simulink model "UNCCModel"  (R2018b)
settings: Solver=ode4  StartTime=0.0  StopTime=Inf  FixedStep=0.025  RelTol=1e-3  EnableMultiTasking=on
PreLoadFcn:
  | preLoadCallback
StartFcn:
  | startCallback
StopFcn:
  | stopCallback
model workspace (MAT data in the model file):
  Ts = 0.025
undefined symbols (not defined in the file or in its folder): acA2000, Ace, Basler, Freerun_FIX_YAW, PoCL
libraries: slrtlib x3, xpcbitflowlib x3, xpcvideoutillib x2, xpcobsoletelib x1, xpcrtudplib x1
(part 1 of 3)
settings Model: xpc_rtwmakecfg_data=_jpeg__bitflow_  sg_rtwmakecfg_data=_bitflow_  SimulationMode=external  Creator=gweast  LastModifiedBy=MAE-NCSUCORE
settings DataIOCC: MaxDataPoints=40*60*60  SaveFormat=Array  SignalLoggingSaveFormat=ModelDataLogs  SignalLogging=off  DSMLogging=off  VisualizeSimOutput=off
settings OptimizationCC: BlockReduction=off  OptimizeBlockIOStorage=off  BufferReuse=off  GlobalBufferReuse=off  ExpressionFolding=off  ExpressionDepthLimit=2147483647  LocalBlockOutputs=off  LifeSpan=inf  SimCompilerOptimization=on  OptimizeDataStoreBuffers=off  BusAssignmentInplaceUpdate=off
settings DebuggingCC: UnderspecifiedInitializationDetection=Classic  MergeDetectMultiDrivingBlocksExec=none  SolverPrmCheckMsg=warning  InheritedTsInSrcMsg=none  FcnCallInpInsideContextMsg=warning  AllowSymbolicDim=off  StateNameClashWarn=warning  LibraryContextMissingDiagnostic=none  SFUnexpectedBacktrackingDiag=warning  SFNoUnconditionalDefaultTransitionDiag=warning  SFExecutionAtInitializationDiag=none
settings HardwareCC: ProdBitPerPointer=32  ProdBitPerSizeT=32  ProdBitPerPtrDiffT=32  ProdLargestAtomicFloat=None  ProdWordSize=32  ProdLongLongMode=on  ProdHWDeviceType=Generic->32-bit x86 compatible  TargetBitPerLong=64  TargetBitPerPointer=64  TargetIntDivRoundTo=Zero  TargetEndianess=LittleEndian  TargetWordSize=64  TargetHWDeviceType=Intel->x86-64
settings ModelReferenceCC: UpdateModelReferenceTargets=Force  PropagateSignalLabelsOutOfModel=off
settings SFSimCC: SimUseLocalCustomCode=off
settings RTWCC: SystemTargetFile=slrt.tlc  TLCOptions=-axPCModelStackSizeKB=512  TemplateMakefile=slrt_default_tmf  Description=Simulink Real-Time  GenerateReport=on  RTWUseLocalCustomCode=off  CodeExecutionProfiling=on  RTWCompilerOptimization=on
settings CodeAppCC: StateflowObjectComments=on
settings SimulinkRealTimeCC: PreserveStateflowLocalDataDimensions=off  RL32LogBufSizeModifier=32400000  xPCRL32EventNumber=50000  xPCisModelTimeout=off  xPCModelTimeoutSecs=30
settings ConfigComp: CovMetricSettings=dw  CovHtmlReporting=on  CovSaveCumulativeToWorkspaceVar=on  CovSaveSingleToWorkspaceVar=on  CovExternalEMLEnable=off

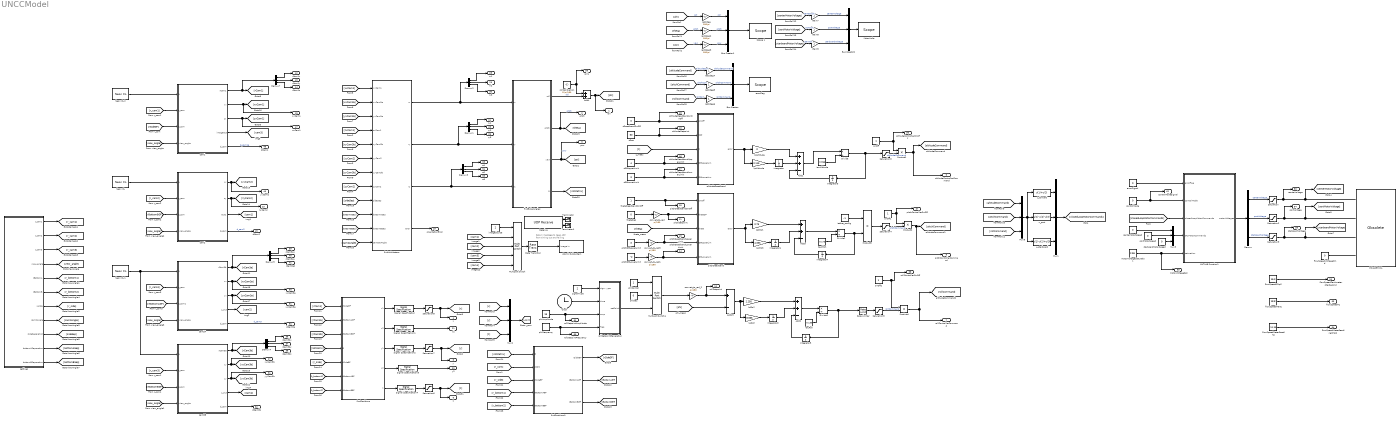
== system UNCCModel ==
  note: Return message to keep ARP
      | from timing out and failing
  Add1 : Sum  Inputs=++-
  Add19 : Sum  Inputs=+-
  Add2 : Sum  Inputs=++-
  Add3 : Sum  Inputs=++-
  Add4 : Sum
  Atomic Subsystem : Subsystem  TreatAsAtomicUnit=on  SystemSampleTime=Ts*3
  Bus Creator : BusCreator  Inputs=3
  Bus Creator1 : BusCreator  Inputs=3
  Bus Creator2 : BusCreator  Inputs=3
  Clock : Clock
  Demux{,1..5,7} (7 alike) : Demux  Outputs=3
  Divide : Product  Inputs=*/
  Divide1 : Product  Inputs=*/
  Divide2 : Product  Inputs=*/
  Gain7 : Gain
  Gain8 : Gain
  Gain9 : Gain
  Integrator{,1..5} (6 alike) : Integrator  InitialCondition=0.001
  MATLAB Function1 : MATLAB Function  TreatAsAtomicUnit=on
  "MotorVolts " : slrtlib/Displays and Logging/Scope   Tag=Motor Volts  Priority=2  scopeno=2  scopetype=Target  autostart=on  viewmode=Graphical rolling  formatstr='%15.6f'  grid=on  ylimits=[0,4]  nosamples=400  noprepostsamples=0  interleave=1  triggermode=FreeRun  triggersignal=1  trigsignalfromport=off  triggerlevel=0.0  triggerslope=Either  triggerscope=1  triggersample=0  filename=data.dat  mode=Lazy  writesize=512  autorestart=off  dynamicfilemode=off  maxwritefilesize=512*1024^2
  Multiport Switch : MultiPortSwitch  DataPortOrder=Zero-based contiguous  Inputs=4  zeroidx=on
  Multiport Switch4 : MultiPortSwitch  Inputs=2
  Mux{1..3,8} (4 alike) : Mux  Inputs=3
  "Neon CL " : xpcbitflowlib/Neon CL   camerapath=Basler-Ace-acA2000-340km-PoCL-3Tap-Freerun_FIX - ROLL.r64  r64=CAMERA  sampletime=-1  slot=[7,12]  make=Basler  model=acA2000-340km  mode=3 tap, 8-bits, 2040x1088 PoCL Free running  owner=BitFlow  revision=1  modelcomp=0  revcomp=0  aqtimeout=61440  format=1  flashmux=Mux_2TOEP  flashdcc=DCC  pixbitdepth=8  xsize=2040  ysize=1088  xstart=0  ystart=0  dx=2040  dy=1088  expmod="[0  0]"  config="[4294967295         128;4294967295           0;4294967295         512;4294967295           0;4294967295           0;4294967295           0;4294967295      262144;4294967295           0;4294967295           0;4294967295           0;4294967295     4195324;4294967295           0;4294967295           0;4294967295  4294967295;4294967295           0;4294967295           0;4294967295           0;4294967295    16777215;4294967295        1088;4294967295           0;4294967295           0;4294967295    16777215;4294967295           0;4294967295           0;4294967295           0;4294967295           0;4294967295           0;4294967295           0]"  ctab="[6      0     16      1  36880      2     16     96     18     97     16  32768      0]"  qtabmodel="[1   2040  65536]"  trigmode=0  baud=1  bytewidth=4  parity=1  stopbits=1  command="\"\""  response=0  comments=|
      | Three tap camera, 
      | Acquistion acquires 24 bits per clock, 
      | DMA works as 8-bit data
      | Set XSIZE = 3 * ACPL
      settings: SourceProductName=Simulink Real-Time: Speedgoat I/O Driver Library
  Neon CL 1 : xpcbitflowlib/Neon CL   camerapath=Basler-Ace-acA2000-340km-PoCL-3Tap-Freerun_FIX_YAW.r64  r64=CAMERA  sampletime=-1  slot=[4,12]  make=Basler  model=acA2000-340km  mode=3 tap, 8-bits, 2040x1088 PoCL Free running  owner=BitFlow  revision=1  modelcomp=0  revcomp=0  aqtimeout=61440  format=1  flashmux=Mux_2TOEP  flashdcc=DCC  pixbitdepth=8  xsize=2040  ysize=1088  xstart=0  ystart=0  dx=2040  dy=1088  expmod="[0  0]"  config="[4294967295         128;4294967295           0;4294967295         512;4294967295           0;4294967295           0;4294967295           0;4294967295      262144;4294967295           0;4294967295           0;4294967295           0;4294967295     4195324;4294967295           0;4294967295           0;4294967295  4294967295;4294967295           0;4294967295           0;4294967295           0;4294967295     4958209;4294967295        1088;4294967295           0;4294967295           0;4294967295  2164260863;4294967295           0;4294967295           0;4294967295           0;4294967295           0;4294967295     4958208;4294967295           0]"  ctab="[6      0     16      1  36880      2     16     96     18     97     16  32768      0]"  qtabmodel="[1   2040  65536]"  trigmode=0  baud=1  bytewidth=4  parity=1  stopbits=1  command="\"\""  response=0  comments=|
      | Three tap camera, 
      | Acquistion acquires 24 bits per clock, 
      | DMA works as 8-bit data
      | Set XSIZE = 3 * ACPL
      settings: SourceProductName=Simulink Real-Time: Speedgoat I/O Driver Library
  Neon CL 2 : xpcbitflowlib/Neon CL   camerapath=Basler-Ace-acA2000-340km-PoCL-3Tap-Freerun_FIX - PITCH.r64  r64=CAMERA  sampletime=-1  slot=[13,12]  make=Basler  model=acA2000-340km  mode=3 tap, 8-bits, 2040x1088 PoCL Free running  owner=BitFlow  revision=1  modelcomp=0  revcomp=0  aqtimeout=61440  format=1  flashmux=Mux_2TOEP  flashdcc=DCC  pixbitdepth=8  xsize=2040  ysize=1088  xstart=0  ystart=0  dx=2040  dy=1088  expmod="[0  0]"  config="[4294967295         128;4294967295           0;4294967295         512;4294967295           0;4294967295           0;4294967295           0;4294967295      262144;4294967295           0;4294967295           0;4294967295           0;4294967295     4195324;4294967295           0;4294967295           0;4294967295  4294967295;4294967295           0;4294967295           0;4294967295           0;4294967295     7528449;4294967295        1088;4294967295           0;4294967295           0;4294967295           0;4294967295           0;4294967295           0;4294967295           0;4294967295           0;4294967295     7528448;4294967295           0]"  ctab="[6      0     16      1  36880      2     16     96     18     97     16  32768      0]"  qtabmodel="[1   2040  65536]"  trigmode=0  baud=1  bytewidth=4  parity=1  stopbits=1  command="\"\""  response=0  comments=|
      | Three tap camera, 
      | Acquistion acquires 24 bits per clock, 
      | DMA works as 8-bit data
      | Set XSIZE = 3 * ACPL
      settings: SourceProductName=Simulink Real-Time: Speedgoat I/O Driver Library
  PCI-6259 DA : xpcobsoletelib/Obsolete
      settings: SourceProductName=Simulink Real-Time  SourceProductBaseCode=XP
  Product{1..4} (4 alike) : Product
  Rate Limiter : RateLimiter  RisingSlewLimit=20  FallingSlewLimit=-20  SampleTimeMode=inherited
  Rate Transition : RateTransition
  Receive : xpcrtudplib/UDP Receive  ipAddressVal=Use host-target connection  localPort=25005  rcvWidth=1  rcvFmAny=off  fmAddress=10.10.10.10  rcvMulticast=off  multicastAddress=[]  maxUDPQueue=8  sampleTime=-1
      settings: SourceProductName=Simulink Real-Time
  Saturation : Saturate  UpperLimit=3.3  LowerLimit=0
  Saturation2 : Saturate  UpperLimit=3.3  LowerLimit=0
  Saturation3 : Saturate  UpperLimit=1.65  LowerLimit=-1.65
  Saturation4 : Saturate  UpperLimit=1.65  LowerLimit=-1.65
  Saturation5 : Saturate  UpperLimit=1.65  LowerLimit=-1.65
  Saturation6 : Saturate  UpperLimit=90  LowerLimit=10
  Saturation7 : Saturate  UpperLimit=50  LowerLimit=-50
  Saturation8 : Saturate  UpperLimit=100  LowerLimit=-10
  Saturation9 : Saturate  UpperLimit=3.3  LowerLimit=0
  Scope 1 : slrtlib/Displays and Logging/Scope   scopeno=1  scopetype=Target  autostart=on  viewmode=Graphical rolling  formatstr='%15.6f'  grid=on  ylimits=[-45,45]  nosamples=400  noprepostsamples=0  interleave=1  triggermode=FreeRun  triggersignal=1  trigsignalfromport=off  triggerlevel=0.0  triggerslope=Either  triggerscope=1  triggersample=0  filename=data.dat  mode=Lazy  writesize=512  autorestart=off  dynamicfilemode=off  maxwritefilesize=512*1024^2
  Signal Specification{,1..4} (5 alike) : SignalSpecification  Dimensions=1
  Terminator : Terminator
  Terminator1 : Terminator
  altitudeDeadband : MATLAB Function  TreatAsAtomicUnit=on
  cam1 : Subsystem
  cam2 : Subsystem
  cam3A : Subsystem
  cam3B : Subsystem
  centerMotorSpeed : Constant  Value=0
  controlMode : Constant  Value=0
  convert_to_rad : Gain  Gain=pi/180
  convert_to_rad1 : Gain  Gain=pi/180
  convert_to_rad3 : Gain  Gain=pi/180
  convert_to_rad_2 : Gain  Gain=pi/180
  errorFlag : slrtlib/Displays and Logging/Scope   Tag=Motor Volts  Priority=2  scopeno=4  scopetype=Target  autostart=on  viewmode=Graphical rolling  formatstr='%15.6f'  grid=on  ylimits=[-2,2]  nosamples=400  noprepostsamples=0  interleave=1  triggermode=FreeRun  triggersignal=1  trigsignalfromport=off  triggerlevel=0.0  triggerslope=Either  triggerscope=1  triggersample=0  filename=data.dat  mode=Lazy  writesize=512  autorestart=off  dynamicfilemode=off  maxwritefilesize=512*1024^2
  errorSignal : Constant  Value=0
  findEulerAngles : MATLAB Function  TreatAsAtomicUnit=on
  findPositions : MATLAB Function  TreatAsAtomicUnit=on
  findPositions1 : MATLAB Function  TreatAsAtomicUnit=on
  findUnitVectors : MATLAB Function  TreatAsAtomicUnit=on
  flowSpeedCMpS : Constant  Value=16.3
  flowSpeedHertz : Constant  Value=18.8
  flowSpeedMeterReading : Constant  Value=20.39
  flowSpeedVoltageCmd : Constant  Value=0
  imageSource : Constant  Value=2
  kdAltitude : Gain  Gain=0
  kdPitch : Gain  Gain=0.75
  kdRoll : Gain  Gain=2.250
  kpAltitude : Gain  Gain=0.115
  kpPitch : Gain  Gain=4.333
  kpRoll : Gain  Gain=8.666
  motorVoltageSaturation : Constant  Value=2.56
  onOff : Constant
  onOff1 : Constant
  onOff2 : Constant
  phiAmplitude : Constant  Value=15
  phiControl : Constant
  phiDes : Constant  Value=0
  phiFrequency : Constant  Value=1/6.875
  pitchDBLowerLimit : Constant  Value=-2
  pitchDBUpperLimit : Constant  Value=3
  pitchDeadband : MATLAB Function  TreatAsAtomicUnit=on
  portMotorSpeed : Constant  Value=0
  rad2deg : Gain  Gain=180/pi
  rad2deg2 : Gain  Gain=180/pi
  rad2deg3 : Gain  Gain=180/pi
  rad2deg4 : Gain
  "rad2deg5 " : Gain
  rad2deg6 : Gain
  rollCalibration : Constant  Value=5*pi/180
  rollSetpointGeneration : MATLAB Function  TreatAsAtomicUnit=on
  settings : Subsystem
  signalType : Constant  Value=2
  starboardMotorSpeed : Constant  Value=0
  tauAltitude : Constant  Value=0.866
  tauPitch : Constant  Value=0.173
  tauRoll : Constant  Value=0.130
  tether_config : Constant  Value=-1
  thetaDeadbandOnOff : Constant
  thetaDes : Constant  Value=0
  u_forward : Fcn  Expr=u(1)+u(2)
  u_port : Fcn  Expr=u(1)-u(2)-u(3)
  u_starboard : Fcn  Expr=u(1)-u(2)+u(3)
  zDBLowerLimit : Constant  Value=3
  zDBUpperLimit : Constant  Value=4
  zDeadbandOnOff : Constant  Value=0
  zDes : Constant  Value=50
  roll : Outport
  pitch : Outport  Port=2
  yaw : Outport  Port=3
  x : Outport  Port=4
  y : Outport  Port=5
  z : Outport  Port=6
  rollControllerCommand : Outport  Port=7
  pitchControllerCommand : Outport  Port=8
  altitudeControllerCommand : Outport  Port=9
  altitudeSetpoint : Outport  Port=10
  pitchSetpoint : Outport  Port=11
  rollSetpoint : Outport  Port=12
  pitchDeadbandUpperLimit : Outport  Port=13
  pitchDeadbandLowerLimit : Outport  Port=14
  pitchDeadbandOnOff : Outport  Port=15
  altitudeDeadbandUpperLimit : Outport  Port=16
  altitudeDeadbandLowerLimit : Outport  Port=17
  altitudeDeadbandonOnOff : Outport  Port=18
  orientationError : Outport  Port=19
  flowSpeedCentimetersPerSecond : Outport  Port=20
  x2 : Outport  Port=21
  y2 : Outport  Port=22
  zyCam2 : Outport  Port=23
  ry1 : Outport  Port=24
  ry2 : Outport  Port=25
  ry3 : Outport  Port=26
  xyCam3b : Outport  Port=27
  rx1 : Outport  Port=28
  rx2 : Outport  Port=29
  rx3 : Outport  Port=30
  yyCam3b : Outport  Port=31
  dCam3b : Outport  Port=32
  rz1 : Outport  Port=33
  rz2 : Outport  Port=34
  rz3 : Outport  Port=35
  rCam3bx : Outport  Port=36
  rCam3by : Outport  Port=37
  rCam3bz : Outport  Port=38
  rCam3ax : Outport  Port=39
  rCam3ay : Outport  Port=40
  rCam3az : Outport  Port=41
  rCam1x : Outport  Port=42
  rCam1y : Outport  Port=43
  rCam1z : Outport  Port=44
  yyCam2 : Outport  Port=45
  xxCam1 : Outport  Port=46
  zxCam1 : Outport  Port=47
  dCam1 : Outport  Port=48
  dCam2 : Outport  Port=49
  xxCam3a : Outport  Port=50
  yxCam3a : Outport  Port=51
  dCam3a : Outport  Port=52
  centerVoltage : Outport  Port=53
  portVoltage : Outport  Port=54
  starboardVoltage : Outport  Port=55
  altitudeControllerOnOff : Outport  Port=56
  pitchControllerOnOff : Outport  Port=57
  rollControllerOnOff : Outport  Port=58
  roll1 : Outport  Port=59
  rollSetpointFrequency : Outport  Port=60
  rollSetpointAmplitude : Outport  Port=61
  controlModeSignal : Outport  Port=62
  flowSpeedHz : Outport  Port=63
  flowSpeedMeterReadingCMpS : Outport  Port=64
  motorVoltageSat : Outport  Port=65
  wires:
  controlMode/1 -> controlModeSignal/1, MATLAB Function1/2(controlMode)
  [phi] -> Add19/2
  [theta] -> pitchDeadband/3(theta)
  cam1/1(rCam1) -> [rCam1], Demux7/1
  cam3A/1(rCam3b) -> Demux5/1, [rCam3a]
  Demux/3 -> Saturation9/1  "starboardVoltage"
  Neon CL 1/1 -> cam3B/1("u "), cam3A/1(u)
  cam1/2(xx) -> xxCam1/1, [xxCam1]
  cam1/3(zx) -> zxCam1/1, [zxCam1]
  cam3A/3(yx) -> yxCam3a/1, [yxCam3a]
  findEulerAngles/2(pitch) -> [theta], pitch/1  "pitch"
  findEulerAngles/3(yaw) -> [psi], yaw/1  "yaw"
  convert_to_rad_2/1 -> Add19/1, rollSetpoint/1
  tether_config/1 -> Product3/1
  Product3/1 -> Saturation4/1
  cam3B/2(xy) -> xyCam3b/1, [xyCam3b]
  cam3B/3(yy) -> yyCam3b/1, [yyCam3b]
  cam2/1(yy) -> yyCam2/1, [yyCam2]
  cam2/2(zy) -> zyCam2/1, [zyCam2]
  Neon CL 2/1 -> cam1/1("u ")
  cam3B/4(u_out) -> [cam4]
  cam2/3(Out1) -> [cam1]
  "Neon CL "/1 -> cam2/1("u ")
  cam3A/4("u_out ") -> [cam2]
  settings/1(r_cam1) -> [r_cam1]
  settings/2("r_cam2 ") -> [r_cam2]
  settings/3(r_cam3) -> [r_cam3]
  [r_cam1] -> cam1/2(r_cam)
  [r_cam3] -> cam3B/2(r_cam)
  [r_cam2] -> cam2/2(r_cam)
  [r_cam3] -> cam3A/2(r_cam)
  [rBottomBGF] -> cam3B/3("r_com ")
  [rBottomBGF] -> cam2/3("r_com ")
  [rBottomAGF] -> cam3A/3(r_com1)
  [rSideGF] -> cam1/3("r_com ")
  cam3B/5(d_cam) -> dCam3b/1
  settings/4(view_angle) -> [view_angle]
  [view_angle] -> cam1/4(view_angle)
  [view_angle] -> cam3B/4(view_angle)
  [view_angle] -> cam2/4(view_angle)
  [view_angle] -> cam3A/4(view_angle)
  cam1/4(imageOut) -> [cam3]
  phiAmplitude/1 -> rollSetpointAmplitude/1, rollSetpointGeneration/3(amp)
  phiFrequency/1 -> rollSetpointFrequency/1, rollSetpointGeneration/4(freq)
  Multiport Switch4/1 -> convert_to_rad_2/1
  rollSetpointGeneration/1(setPoint) -> Multiport Switch4/3
  phiDes/1 -> Multiport Switch4/2
  phiControl/1 -> Multiport Switch4/1
  thetaDes/1 -> convert_to_rad/1
  Clock/1 -> rollSetpointGeneration/2(time)
  portMotorSpeed/1 -> Mux3/2
  Mux3/1 -> MATLAB Function1/4(GUIMotorCommands)
  signalType/1 -> rollSetpointGeneration/1(signalType)
  Rate Limiter/1 -> Saturation5/1
  zDes/1 -> altitudeDeadband/2(zSP), altitudeSetpoint/1
  u_forward/1 -> Mux1/1
  u_port/1 -> Mux1/2
  u_starboard/1 -> Mux1/3
  [closedLoopMotorCommands] -> MATLAB Function1/3(closedLoopMotorCommands)
  centerMotorSpeed/1 -> Mux3/1
  starboardMotorSpeed/1 -> Mux3/3
  [psi] -> rad2deg3/1  "yaw"
  [theta] -> rad2deg2/1  "pitch"
  [phi] -> rad2deg/1  "roll"
  [z] -> Mux2/3
  [y] -> Mux2/2
  [x] -> Mux2/1
  Saturation6/1 -> z/1, [z]
  Saturation7/1 -> [y], y/1
  Saturation8/1 -> x/1, [x]
  [rollCommand] -> Mux8/3
  [pitchCommand] -> Mux8/2
  [altitudeCommand] -> Mux8/1
  Divide/1 -> Integrator3/1, Saturation3/1
  Divide1/1 -> Integrator4/1, Product3/2
  MATLAB Function1/1(motorVoltages) -> Demux/1
  Demux/2 -> Saturation2/1  "portVoltage"
  Demux/1 -> Saturation/1  "centerVoltage"
  Bus Creator2/1 -> "MotorVolts "/1
  settings/5(rBottomA) -> [r_bottom1]
  settings/7(r_side) -> [r_side]
  convert_to_rad/1 -> pitchSetpoint/1, pitchDeadband/2(thetaSP)
  pitchDBUpperLimit/1 -> convert_to_rad3/1
  convert_to_rad3/1 -> pitchDeadband/4(DBUpperLim), pitchDeadbandUpperLimit/1
  errorSignal/1 -> MATLAB Function1/1(errorFlag)
  pitchDBLowerLimit/1 -> convert_to_rad1/1
  convert_to_rad1/1 -> pitchDeadband/5(DBLowerLim), pitchDeadbandLowerLimit/1
  thetaDeadbandOnOff/1 -> pitchDeadbandOnOff/1, pitchDeadband/1(onOff)
  [z] -> altitudeDeadband/3(z)
  zDeadbandOnOff/1 -> altitudeDeadbandonOnOff/1, altitudeDeadband/1(onOff)
  zDBUpperLimit/1 -> altitudeDeadbandUpperLimit/1, altitudeDeadband/4(DBUpperLim)
  zDBLowerLimit/1 -> altitudeDeadbandLowerLimit/1, altitudeDeadband/5(DBLowerLim)
  [zyCam2] -> findUnitVectors/8(zyCam2)
  [xxCam1] -> findUnitVectors/1(xxCam1)
  [zxCam1] -> findUnitVectors/4(zxCam1)
  [xxCam3a] -> findUnitVectors/2(xxCam3a)
  [xyCam3b] -> findUnitVectors/5(xyCam3b)
  [yxCam3a] -> findUnitVectors/3(yxCam3a)
  [yyCam3b] -> findUnitVectors/7(yyCam3b)
  [yyCam2] -> findUnitVectors/6(yyCam2)
  [cam2Angle] -> findUnitVectors/12(cameraAngle)
  settings/8(cam2Angle) -> [cam2Angle]
  findUnitVectors/4(error) -> orientationError/1
  settings/6(rBottomB) -> [r_bottom2]
  cam3B/1(rCam3a) -> Demux4/1, [rCam3b]
  [rCam1] -> findPositions/1(rSideGF)
  [rCam3a] -> findPositions/2(rBottomAGF)
  [rCam3b] -> findPositions/3(rBottomBGF)
  [r_side] -> findPositions/5(rSideBF)
  [r_bottom1] -> findPositions/6(rBottomABF)
  [r_bottom2] -> findPositions/7(rBottomBBF)
  [bottomBSep] -> findUnitVectors/11(bottomBSep)
  [bottomASep] -> findUnitVectors/10(bottomASep)
  [sideSep] -> findUnitVectors/9(sideSep)
  settings/9(sideSeparation) -> [sideSep]
  settings/10(bottomASeparation) -> [bottomASep]
  settings/11(bottomBSeparation) -> [bottomBSep]
  [rotMatrix] -> findPositions/4(R)
  Rate Transition/1 -> Atomic Subsystem/1(Image In)
  Receive/1 -> Terminator/1
  Receive/2 -> Terminator1/1
  imageSource/1 -> Multiport Switch/1
  [cam1] -> Multiport Switch/2
  [cam3] -> Multiport Switch/4
  [cam2] -> Multiport Switch/3
  Multiport Switch/1 -> Rate Transition/1
  [cam4] -> Multiport Switch/5
  findEulerAngles/4(R) -> [rotMatrix]
  flowSpeedCMpS/1 -> flowSpeedCentimetersPerSecond/1
  kpAltitude/1 -> Integrator/1
  altitudeDeadband/1(error) -> kpAltitude/1, kdAltitude/1
  kdAltitude/1 -> Add1/1
  Integrator/1 -> Add1/2
  Add1/1 -> Divide/1
  tauAltitude/1 -> Divide/2
  Integrator3/1 -> Add1/3
  cam1/5(d_cam) -> dCam1/1  "d_cam1a"
  cam2/4(d_cam) -> dCam2/1  "d_cam2"
  cam3A/5(d_cam) -> dCam3a/1  "d_cam3"
  Bus Creator1/1 -> Scope 1/1
  Mux1/1 -> [closedLoopMotorCommands]
  pitchDeadband/1(error) -> kdPitch/1, kpPitch/1
  kpPitch/1 -> Integrator1/1
  Integrator1/1 -> Add3/2
  kdPitch/1 -> Add3/1
  Add3/1 -> Divide1/1
  tauPitch/1 -> Divide1/2
  Integrator4/1 -> Add3/3
  Add19/1 -> kpRoll/1, kdRoll/1
  kpRoll/1 -> Integrator2/1
  Integrator2/1 -> Add2/2
  kdRoll/1 -> Add2/1
  Add2/1 -> Divide2/1
  tauRoll/1 -> Divide2/2
  Integrator5/1 -> Add2/3
  Divide2/1 -> Integrator5/1, Rate Limiter/1
  Mux8/1 -> u_starboard/1, u_forward/1, u_port/1
  Bus Creator/1 -> errorFlag/1
  findPositions/1(x1) -> Signal Specification/1
  findPositions/5(z) -> Signal Specification4/1
  findPositions/3(y1) -> Signal Specification2/1
  findPositions/2(x2) -> Signal Specification1/1
  findPositions/4(y2) -> Signal Specification3/1
  rad2deg/1 -> Bus Creator1/1  "roll"
  rad2deg2/1 -> Bus Creator1/2  "pitch"
  rad2deg3/1 -> Bus Creator1/3  "yaw"
  [altitudeCommand] -> rad2deg4/1  "altitudeCom"
  [pitchCommand] -> "rad2deg5 "/1  "pitchCom"
  [rollCommand] -> rad2deg6/1  "rollCom"
  rad2deg4/1 -> Bus Creator/1  "altitudeCommand"
  "rad2deg5 "/1 -> Bus Creator/2  "pitchCommand"
  rad2deg6/1 -> Bus Creator/3  "rollCommand"
  [centerMotorVoltage] -> Gain7/1  "centerVolt"
  [portMotorVoltage] -> Gain8/1  "portVolt"
  [starboardMotorVoltage] -> Gain9/1  "starVolt"
  Gain7/1 -> Bus Creator2/1  "centerVoltage"
  Gain8/1 -> Bus Creator2/2  "portVoltage"
  Gain9/1 -> Bus Creator2/3  "starboardVoltage"
  Demux1/1 -> ry1/1
  Demux1/2 -> ry2/1
  Demux1/3 -> ry3/1
  Demux2/1 -> rx1/1
  Demux2/2 -> rx2/1
  Demux2/3 -> rx3/1
  Demux3/1 -> rz1/1
  Demux3/2 -> rz2/1
  Demux3/3 -> rz3/1
  Demux4/1 -> rCam3bx/1
  Demux4/2 -> rCam3by/1
  Demux4/3 -> rCam3bz/1
  Demux5/1 -> rCam3ax/1
  Demux5/2 -> rCam3ay/1
  Demux5/3 -> rCam3az/1
  Demux7/1 -> rCam1x/1
  Demux7/2 -> rCam1y/1
  Demux7/3 -> rCam1z/1
  cam3A/2(xx) -> xxCam3a/1, [xxCam3a]
  Saturation/1 -> centerVoltage/1, [centerMotorVoltage]
  Saturation2/1 -> portVoltage/1, [portMotorVoltage]
  Saturation9/1 -> starboardVoltage/1, [starboardMotorVoltage]
  Saturation3/1 -> Product1/2  "altitudeCommand"
  Product1/1 -> altitudeControllerCommand/1, [altitudeCommand]
  onOff/1 -> altitudeControllerOnOff/1, Product1/1
  Saturation4/1 -> Product2/2  "pitchCommand"
  Product2/1 -> pitchControllerCommand/1, [pitchCommand]
  onOff1/1 -> pitchControllerOnOff/1, Product2/1
  Saturation5/1 -> Product4/2  "rollCommand"
  Product4/1 -> rollControllerCommand/1, [rollCommand]
  onOff2/1 -> rollControllerOnOff/1, Product4/1
  [r_com] -> findPositions1/2(rCOM)
  [r_side] -> findPositions1/3(rSideBF)
  [r_bottom1] -> findPositions1/4(rBottomABF)
  [r_bottom2] -> findPositions1/5(rBottomBBF)
  findPositions1/1(rSideGF) -> [rSideGF]
  findPositions1/2(rBottomAGF) -> [rBottomAGF]
  findPositions1/3(rBottomBGF) -> [rBottomBGF]
  [rotMatrix] -> findPositions1/1(R)
  Add4/1 -> roll/1, [phi]
  findEulerAngles/1(roll) -> Add4/2  "roll"
  rollCalibration/1 -> roll1/1, Add4/1
  Signal Specification/1 -> Saturation8/1
  Signal Specification1/1 -> x2/1
  Signal Specification2/1 -> Saturation7/1
  Signal Specification3/1 -> y2/1
  Signal Specification4/1 -> Saturation6/1
  Mux2/1 -> [r_com]
  findUnitVectors/1(rx) -> Demux2/1, findEulerAngles/1(rx)
  findUnitVectors/2(ry) -> Demux1/1, findEulerAngles/2(ry)
  findUnitVectors/3(rz) -> Demux3/1, findEulerAngles/3(rz)
  motorVoltageSaturation/1 -> motorVoltageSat/1, MATLAB Function1/5(saturation)
  flowSpeedHertz/1 -> flowSpeedHz/1
  flowSpeedMeterReading/1 -> flowSpeedMeterReadingCMpS/1
  flowSpeedVoltageCmd/1 -> ?

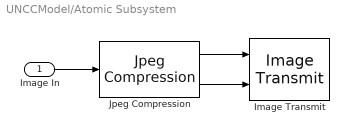
== system UNCCModel/Atomic Subsystem ==
  Image In : Inport
  Image Transmit : xpcvideoutillib/Image Transmit  ipAddress=255.255.255.255  ipPort=25000  localPort=-1  vblLen=on  maxpacket=40*1024  sampletime=-1
      settings: SourceProductName=Simulink Real-Time  SourceProductBaseCode=XP
  Jpeg Compression : xpcvideoutillib/Jpeg Compression  quality=35  cspace=Grayscale  isig=One multidimensional signal  maxsize=2040*1088  length=on
      settings: SourceProductName=Simulink Real-Time  SourceProductBaseCode=XP
  wires:
  Jpeg Compression/1 -> Image Transmit/1
  Jpeg Compression/2 -> Image Transmit/2
  Image In/1 -> Jpeg Compression/1

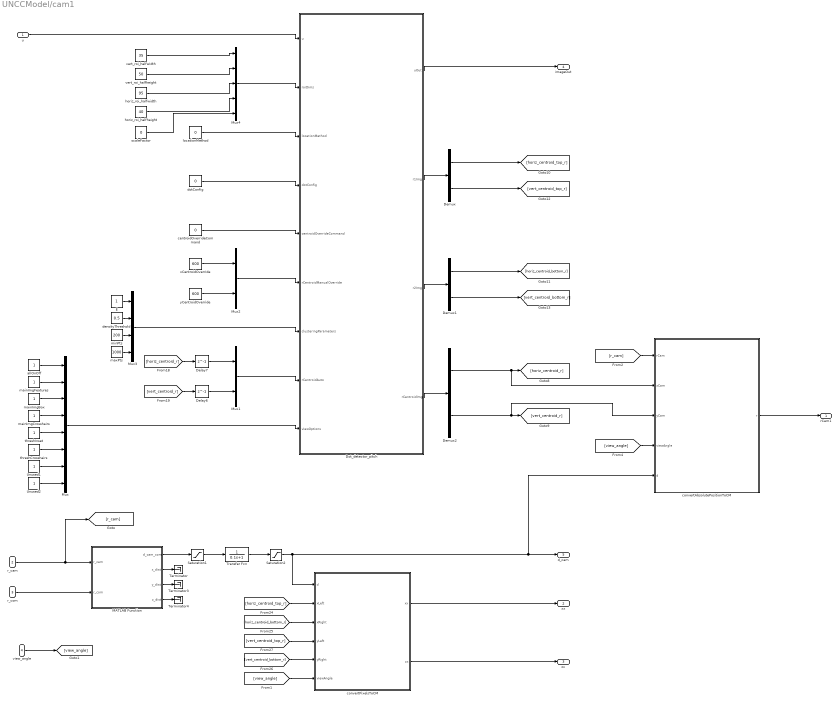
== system UNCCModel/cam1 ==
  "u " : Inport
  r_cam : Inport  Port=2
  "r_com " : Inport  Port=3
  view_angle : Inport  Port=4
  Delay6 : Delay  DelayLength=1  InitialCondition=800
  Delay7 : Delay  DelayLength=1  InitialCondition=1460
  Demux : Demux  Outputs=2
  Demux1 : Demux  Outputs=2
  Demux2 : Demux  Outputs=2
  Dot_detector_pitch : MATLAB Function  TreatAsAtomicUnit=on
  E : Constant
  MATLAB Function : MATLAB Function  TreatAsAtomicUnit=on
  Mux : Mux  Inputs=8
  Mux1 : Mux  Inputs=2
  Mux2 : Mux  Inputs=2
  Mux3 : Mux
  Mux4 : Mux  Inputs=5
  Saturation1 : Saturate  UpperLimit=200  LowerLimit=1
  Saturation2 : Saturate  UpperLimit=200  LowerLimit=1
  Terminator : Terminator
  Terminator3 : Terminator
  Terminator4 : Terminator
  Transfer Fcn : TransferFcn  Denominator=[0.1 1]
  Unused1 : Constant
  Unused2 : Constant
  allOnOff : Constant
  centroidOverrideCommand : Constant  Value=0
  convertAbsolutePositionToCM : MATLAB Function  TreatAsAtomicUnit=on
  convertPixelsToCM : MATLAB Function  TreatAsAtomicUnit=on
  densityThreshold : Constant  Value=0.5
  dotConfig : Constant  Value=0
  horiz_roi_halfheight : Constant  Value=40
  horiz_roi_halfwidth : Constant  Value=95
  locationMethod : Constant  Value=0
  mainImgBox : Constant
  mainImgCrosshairs : Constant
  mainImgFeatures : Constant
  maxPts : Constant  Value=1000
  minPts : Constant  Value=200
  scaleFactor : Constant  Value=0
  threshCrosshairs : Constant
  threshInset : Constant
  vert_roi_halfheight : Constant  Value=50
  vert_roi_halfwidth : Constant  Value=35
  xCentroidOverride : Constant  Value=600
  yCentroidOverride : Constant  Value=600
  rCam1 : Outport
  xx : Outport  Port=2
  zx : Outport  Port=3
  imageOut : Outport  Port=4
  d_cam : Outport  Port=5
  wires:
  Demux/1 -> [horiz_centroid_top_r]
  Demux1/1 -> [horiz_centroid_bottom_r]
  Demux2/2 -> convertAbsolutePositionToCM/3(yCam), [vert_centroid_r]
  Demux1/2 -> [vert_centroid_bottom_r]
  Demux/2 -> [vert_centroid_top_r]
  [horiz_centroid_r] -> Delay7/1
  [vert_centroid_r] -> Delay6/1
  Mux1/1 -> Dot_detector_pitch/8(rCentroidAuto)
  xCentroidOverride/1 -> Mux2/1
  yCentroidOverride/1 -> Mux2/2
  densityThreshold/1 -> Mux3/2
  minPts/1 -> Mux3/3
  maxPts/1 -> Mux3/4
  Mux3/1 -> Dot_detector_pitch/7(clusteringParameters)
  E/1 -> Mux3/1
  centroidOverrideCommand/1 -> Dot_detector_pitch/5(centroidOverrideCommand)
  locationMethod/1 -> Dot_detector_pitch/3(locationMethod)
  dotConfig/1 -> Dot_detector_pitch/4(dotConfig)
  Dot_detector_pitch/2(r1Img) -> Demux/1
  Dot_detector_pitch/3(r2Img) -> Demux1/1
  Dot_detector_pitch/4(rCentroidImg) -> Demux2/1
  Mux2/1 -> Dot_detector_pitch/6(rCentroidManualOverride)
  Delay7/1 -> Mux1/1
  Delay6/1 -> Mux1/2
  allOnOff/1 -> Mux/1
  mainImgFeatures/1 -> Mux/2
  mainImgBox/1 -> Mux/3
  mainImgCrosshairs/1 -> Mux/4
  threshInset/1 -> Mux/5
  threshCrosshairs/1 -> Mux/6
  Unused1/1 -> Mux/7
  Unused2/1 -> Mux/8
  Mux/1 -> Dot_detector_pitch/9(viewOptions)
  "u "/1 -> Dot_detector_pitch/1(u)
  MATLAB Function/2(x_dist) -> Terminator/1
  MATLAB Function/3(y_dist) -> Terminator3/1
  MATLAB Function/4(z_dist) -> Terminator4/1
  r_cam/1 -> [r_cam], MATLAB Function/1(r_cam)
  "r_com "/1 -> MATLAB Function/2(r_com)
  [horiz_centroid_top_r] -> convertPixelsToCM/2(xLeft)
  [horiz_centroid_bottom_r] -> convertPixelsToCM/3(xRight)
  [vert_centroid_top_r] -> convertPixelsToCM/4(yLeft)
  [vert_centroid_bottom_r] -> convertPixelsToCM/5(yRight)
  convertPixelsToCM/1(xx) -> xx/1
  convertPixelsToCM/2(zx) -> zx/1
  Demux2/1 -> convertAbsolutePositionToCM/2(xCam), [horiz_centroid_r]
  view_angle/1 -> [view_angle]
  [view_angle] -> convertPixelsToCM/6(viewAngle)
  vert_roi_halfwidth/1 -> Mux4/1
  horiz_roi_halfheight/1 -> Mux4/4
  vert_roi_halfheight/1 -> Mux4/2
  horiz_roi_halfwidth/1 -> Mux4/3
  MATLAB Function/1(d_cam_com) -> Saturation1/1
  Saturation1/1 -> Transfer Fcn/1
  Transfer Fcn/1 -> Saturation2/1
  convertAbsolutePositionToCM/1(r) -> rCam1/1
  [r_cam] -> convertAbsolutePositionToCM/1(rCam)
  [view_angle] -> convertAbsolutePositionToCM/4(viewAngle)
  Saturation2/1 -> convertPixelsToCM/1(d), convertAbsolutePositionToCM/5(d), d_cam/1
  Dot_detector_pitch/1(uOut) -> imageOut/1
  Mux4/1 -> Dot_detector_pitch/2(roiDims)
  scaleFactor/1 -> Mux4/5

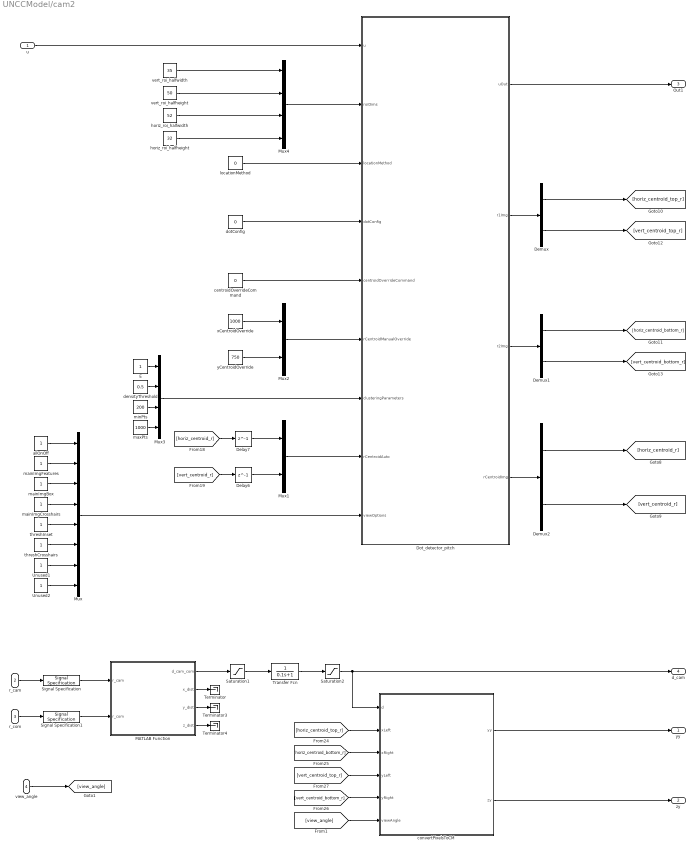
== system UNCCModel/cam2 ==
  "u " : Inport
  r_cam : Inport  Port=2
  "r_com " : Inport  Port=3
  view_angle : Inport  Port=4
  Delay6 : Delay  DelayLength=1  InitialCondition=800
  Delay7 : Delay  DelayLength=1  InitialCondition=1460
  Demux : Demux  Outputs=2
  Demux1 : Demux  Outputs=2
  Demux2 : Demux  Outputs=2
  Dot_detector_pitch : MATLAB Function  TreatAsAtomicUnit=on
  E : Constant
  MATLAB Function : MATLAB Function  TreatAsAtomicUnit=on
  Mux : Mux  Inputs=8
  Mux1 : Mux  Inputs=2
  Mux2 : Mux  Inputs=2
  Mux3 : Mux
  Mux4 : Mux
  Saturation1 : Saturate  UpperLimit=200  LowerLimit=1
  Saturation2 : Saturate  UpperLimit=200  LowerLimit=1
  Signal Specification : SignalSpecification  Dimensions=3
  Signal Specification1 : SignalSpecification  Dimensions=3
  Terminator : Terminator
  Terminator3 : Terminator
  Terminator4 : Terminator
  Transfer Fcn : TransferFcn  Denominator=[0.1 1]
  Unused1 : Constant
  Unused2 : Constant
  allOnOff : Constant
  centroidOverrideCommand : Constant  Value=0
  convertPixelsToCM : MATLAB Function  TreatAsAtomicUnit=on
  densityThreshold : Constant  Value=0.5
  dotConfig : Constant  Value=0
  horiz_roi_halfheight : Constant  Value=32
  horiz_roi_halfwidth : Constant  Value=52
  locationMethod : Constant  Value=0
  mainImgBox : Constant
  mainImgCrosshairs : Constant
  mainImgFeatures : Constant
  maxPts : Constant  Value=1000
  minPts : Constant  Value=200
  threshCrosshairs : Constant
  threshInset : Constant
  vert_roi_halfheight : Constant  Value=50
  vert_roi_halfwidth : Constant  Value=35
  xCentroidOverride : Constant  Value=1000
  yCentroidOverride : Constant  Value=750
  yy : Outport
  zy : Outport  Port=2
  Out1 : Outport  Port=3
  d_cam : Outport  Port=4
  wires:
  Demux/1 -> [horiz_centroid_top_r]
  Demux1/1 -> [horiz_centroid_bottom_r]
  Demux2/2 -> [vert_centroid_r]
  Demux1/2 -> [vert_centroid_bottom_r]
  Demux/2 -> [vert_centroid_top_r]
  [horiz_centroid_r] -> Delay7/1
  [vert_centroid_r] -> Delay6/1
  Mux1/1 -> Dot_detector_pitch/8(rCentroidAuto)
  xCentroidOverride/1 -> Mux2/1
  yCentroidOverride/1 -> Mux2/2
  densityThreshold/1 -> Mux3/2
  minPts/1 -> Mux3/3
  maxPts/1 -> Mux3/4
  Mux3/1 -> Dot_detector_pitch/7(clusteringParameters)
  E/1 -> Mux3/1
  centroidOverrideCommand/1 -> Dot_detector_pitch/5(centroidOverrideCommand)
  locationMethod/1 -> Dot_detector_pitch/3(locationMethod)
  dotConfig/1 -> Dot_detector_pitch/4(dotConfig)
  Dot_detector_pitch/2(r1Img) -> Demux/1
  Dot_detector_pitch/3(r2Img) -> Demux1/1
  Dot_detector_pitch/4(rCentroidImg) -> Demux2/1
  Mux2/1 -> Dot_detector_pitch/6(rCentroidManualOverride)
  Delay7/1 -> Mux1/1
  Delay6/1 -> Mux1/2
  allOnOff/1 -> Mux/1
  mainImgFeatures/1 -> Mux/2
  mainImgBox/1 -> Mux/3
  mainImgCrosshairs/1 -> Mux/4
  threshInset/1 -> Mux/5
  threshCrosshairs/1 -> Mux/6
  Unused1/1 -> Mux/7
  Unused2/1 -> Mux/8
  Mux/1 -> Dot_detector_pitch/9(viewOptions)
  Dot_detector_pitch/1(uOut) -> Out1/1
  "u "/1 -> Dot_detector_pitch/1(u)
  MATLAB Function/2(x_dist) -> Terminator/1
  MATLAB Function/3(y_dist) -> Terminator3/1
  MATLAB Function/4(z_dist) -> Terminator4/1
  r_cam/1 -> Signal Specification/1
  "r_com "/1 -> Signal Specification1/1
  [horiz_centroid_top_r] -> convertPixelsToCM/2(xLeft)
  [horiz_centroid_bottom_r] -> convertPixelsToCM/3(xRight)
  [vert_centroid_top_r] -> convertPixelsToCM/4(yLeft)
  [vert_centroid_bottom_r] -> convertPixelsToCM/5(yRight)
  convertPixelsToCM/1(yy) -> yy/1
  convertPixelsToCM/2(zy) -> zy/1
  Demux2/1 -> [horiz_centroid_r]
  view_angle/1 -> [view_angle]
  [view_angle] -> convertPixelsToCM/6(viewAngle)
  Mux4/1 -> Dot_detector_pitch/2(roiDims)
  vert_roi_halfwidth/1 -> Mux4/1
  horiz_roi_halfheight/1 -> Mux4/4
  vert_roi_halfheight/1 -> Mux4/2
  horiz_roi_halfwidth/1 -> Mux4/3
  MATLAB Function/1(d_cam_com) -> Saturation1/1
  Saturation1/1 -> Transfer Fcn/1
  Transfer Fcn/1 -> Saturation2/1
  Saturation2/1 -> convertPixelsToCM/1(d), d_cam/1
  Signal Specification/1 -> MATLAB Function/1(r_cam)
  Signal Specification1/1 -> MATLAB Function/2(r_com)

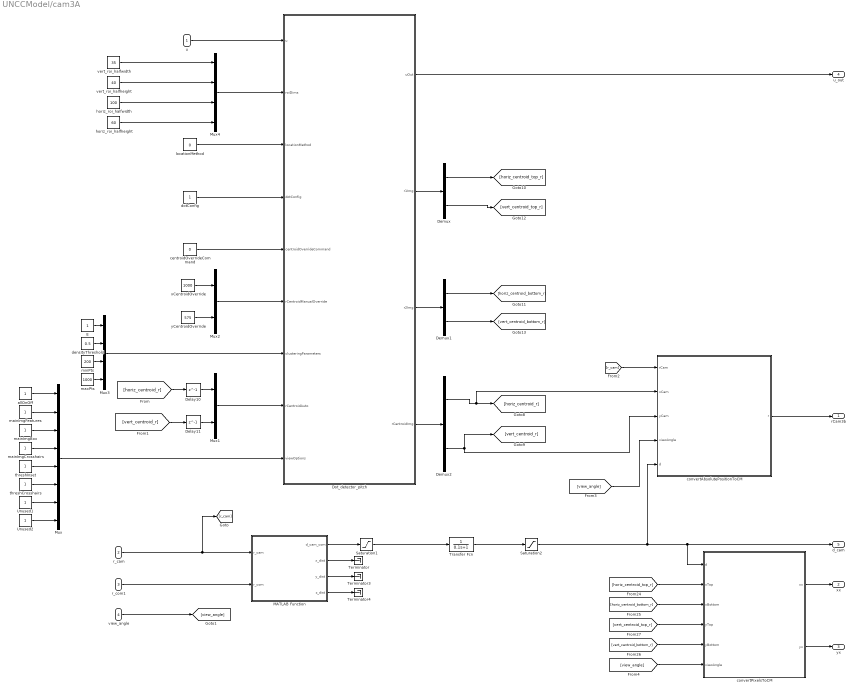
== system UNCCModel/cam3A ==
  u : Inport
  r_cam : Inport  Port=2
  r_com1 : Inport  Port=3
  view_angle : Inport  Port=4
  Delay10 : Delay  DelayLength=1  InitialCondition=1655
  Delay11 : Delay  DelayLength=1  InitialCondition=800
  Demux : Demux  Outputs=2
  Demux1 : Demux  Outputs=2
  Demux2 : Demux  Outputs=2
  Dot_detector_pitch : MATLAB Function  TreatAsAtomicUnit=on
  E : Constant
  MATLAB Function : MATLAB Function  TreatAsAtomicUnit=on
  Mux : Mux  Inputs=8
  Mux1 : Mux  Inputs=2
  Mux2 : Mux  Inputs=2
  Mux3 : Mux
  Mux4 : Mux
  Saturation1 : Saturate  UpperLimit=200  LowerLimit=1
  Saturation2 : Saturate  UpperLimit=200  LowerLimit=1
  Terminator : Terminator
  Terminator3 : Terminator
  Terminator4 : Terminator
  Transfer Fcn : TransferFcn  Denominator=[0.1 1]
  Unused1 : Constant
  Unused2 : Constant
  allOnOff : Constant
  centroidOverrideCommand : Constant  Value=0
  convertAbsolutePositionToCM : MATLAB Function  TreatAsAtomicUnit=on
  convertPixelsToCM : MATLAB Function  TreatAsAtomicUnit=on
  densityThreshold : Constant  Value=0.5
  dotConfig : Constant
  horiz_roi_halfheight : Constant  Value=60
  horiz_roi_halfwidth : Constant  Value=100
  locationMethod : Constant  Value=0
  mainImgBox : Constant
  mainImgCrosshairs : Constant
  mainImgFeatures : Constant
  maxPts : Constant  Value=1000
  minPts : Constant  Value=200
  threshCrosshairs : Constant
  threshInset : Constant
  vert_roi_halfheight : Constant  Value=40
  vert_roi_halfwidth : Constant  Value=35
  xCentroidOverride : Constant  Value=1000
  yCentroidOverride : Constant  Value=575
  rCam3b : Outport
  xx : Outport  Port=2
  yx : Outport  Port=3
  "u_out " : Outport  Port=4
  d_cam : Outport  Port=5
  wires:
  [vert_centroid_r] -> Delay11/1
  [horiz_centroid_r] -> Delay10/1
  allOnOff/1 -> Mux/1
  mainImgFeatures/1 -> Mux/2
  mainImgBox/1 -> Mux/3
  mainImgCrosshairs/1 -> Mux/4
  threshInset/1 -> Mux/5
  threshCrosshairs/1 -> Mux/6
  Unused1/1 -> Mux/7
  Unused2/1 -> Mux/8
  Mux1/1 -> Dot_detector_pitch/8(rCentroidAuto)
  xCentroidOverride/1 -> Mux2/1
  yCentroidOverride/1 -> Mux2/2
  densityThreshold/1 -> Mux3/2
  minPts/1 -> Mux3/3
  maxPts/1 -> Mux3/4
  Mux3/1 -> Dot_detector_pitch/7(clusteringParameters)
  E/1 -> Mux3/1
  centroidOverrideCommand/1 -> Dot_detector_pitch/5(centroidOverrideCommand)
  Mux/1 -> Dot_detector_pitch/9(viewOptions)
  u/1 -> Dot_detector_pitch/1(u)
  locationMethod/1 -> Dot_detector_pitch/3(locationMethod)
  dotConfig/1 -> Dot_detector_pitch/4(dotConfig)
  Dot_detector_pitch/2(r1Img) -> Demux/1
  Dot_detector_pitch/3(r2Img) -> Demux1/1
  Dot_detector_pitch/4(rCentroidImg) -> Demux2/1
  Mux2/1 -> Dot_detector_pitch/6(rCentroidManualOverride)
  Delay10/1 -> Mux1/1
  Delay11/1 -> Mux1/2
  Demux/1 -> [horiz_centroid_top_r]
  Demux/2 -> [vert_centroid_top_r]
  Demux1/1 -> [horiz_centroid_bottom_r]
  Demux1/2 -> [vert_centroid_bottom_r]
  Dot_detector_pitch/1(uOut) -> "u_out "/1
  Demux2/2 -> [vert_centroid_r], convertAbsolutePositionToCM/3(yCam)
  Demux2/1 -> convertAbsolutePositionToCM/2(xCam), [horiz_centroid_r]
  MATLAB Function/2(x_dist) -> Terminator/1
  MATLAB Function/3(y_dist) -> Terminator3/1
  MATLAB Function/4(z_dist) -> Terminator4/1
  [horiz_centroid_top_r] -> convertPixelsToCM/2(xTop)
  [horiz_centroid_bottom_r] -> convertPixelsToCM/3(xBottom)
  [vert_centroid_top_r] -> convertPixelsToCM/4(yTop)
  [vert_centroid_bottom_r] -> convertPixelsToCM/5(yBottom)
  MATLAB Function/1(d_cam_com) -> Saturation1/1
  convertPixelsToCM/2(yx) -> yx/1
  convertPixelsToCM/1(xx) -> xx/1
  [r_cam] -> convertAbsolutePositionToCM/1(rCam)
  convertAbsolutePositionToCM/1(r) -> rCam3b/1
  view_angle/1 -> [view_angle]
  [view_angle] -> convertAbsolutePositionToCM/4(viewAngle)
  [view_angle] -> convertPixelsToCM/6(viewAngle)
  Mux4/1 -> Dot_detector_pitch/2(roiDims)
  vert_roi_halfwidth/1 -> Mux4/1
  horiz_roi_halfheight/1 -> Mux4/4
  vert_roi_halfheight/1 -> Mux4/2
  horiz_roi_halfwidth/1 -> Mux4/3
  Saturation1/1 -> Transfer Fcn/1
  Transfer Fcn/1 -> Saturation2/1
  Saturation2/1 -> convertPixelsToCM/1(d), d_cam/1, convertAbsolutePositionToCM/5(d)
  r_cam/1 -> [r_cam], MATLAB Function/1(r_cam)
  r_com1/1 -> MATLAB Function/2(r_com)

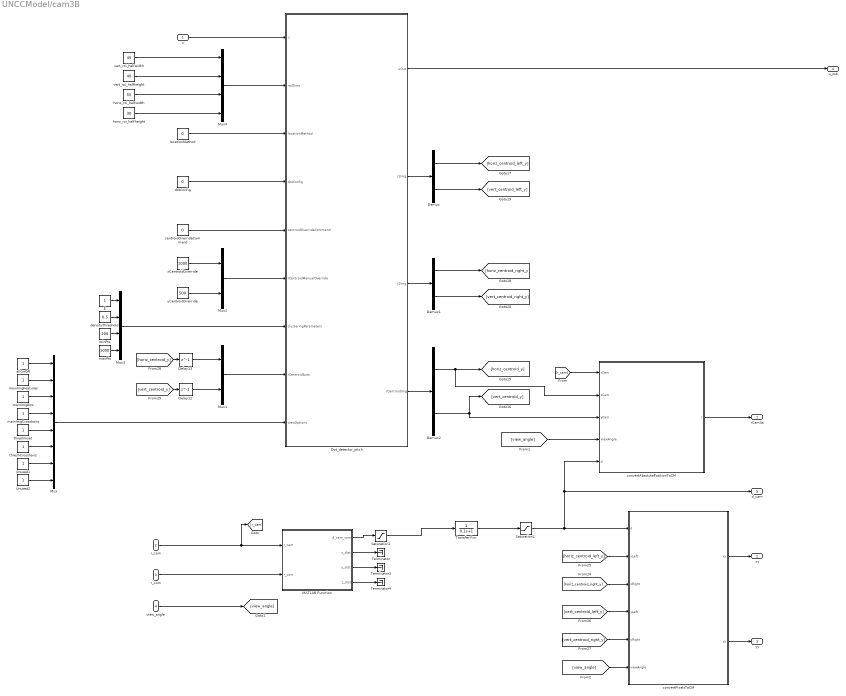
== system UNCCModel/cam3B ==
  "u " : Inport
  r_cam : Inport  Port=2
  "r_com " : Inport  Port=3
  view_angle : Inport  Port=4
  Delay12 : Delay  DelayLength=1  InitialCondition=800
  Delay13 : Delay  DelayLength=1  InitialCondition=1460
  Demux : Demux  Outputs=2
  Demux1 : Demux  Outputs=2
  Demux2 : Demux  Outputs=2
  Dot_detector_pitch : MATLAB Function  TreatAsAtomicUnit=on
  E : Constant
  MATLAB Function : MATLAB Function  TreatAsAtomicUnit=on
  Mux : Mux  Inputs=8
  Mux1 : Mux  Inputs=2
  Mux2 : Mux  Inputs=2
  Mux3 : Mux
  Mux4 : Mux
  Saturation1 : Saturate  UpperLimit=200  LowerLimit=1
  Saturation2 : Saturate  UpperLimit=200  LowerLimit=1
  Terminator : Terminator
  Terminator3 : Terminator
  Terminator4 : Terminator
  Transfer Fcn : TransferFcn  Denominator=[0.1 1]
  Unused1 : Constant
  Unused2 : Constant
  allOnOff : Constant
  centroidOverrideCommand : Constant  Value=0
  convertAbsolutePositionToCM : MATLAB Function  TreatAsAtomicUnit=on
  convertPixelsToCM : MATLAB Function  TreatAsAtomicUnit=on
  densityThreshold : Constant  Value=0.5
  dotConfig : Constant  Value=0
  horiz_roi_halfheight : Constant  Value=30
  horiz_roi_halfwidth : Constant  Value=55
  locationMethod : Constant  Value=0
  mainImgBox : Constant
  mainImgCrosshairs : Constant
  mainImgFeatures : Constant
  maxPts : Constant  Value=1000
  minPts : Constant  Value=200
  threshCrosshairs : Constant
  threshInset : Constant
  vert_roi_halfheight : Constant  Value=40
  vert_roi_halfwidth : Constant  Value=45
  xCentroidOverride : Constant  Value=1000
  yCentroidOverride : Constant  Value=500
  rCam3a : Outport
  xy : Outport  Port=2
  yy : Outport  Port=3
  u_out : Outport  Port=4
  d_cam : Outport  Port=5
  wires:
  [vert_centroid_y] -> Delay12/1
  [horiz_centroid_y] -> Delay13/1
  Mux1/1 -> Dot_detector_pitch/8(rCentroidAuto)
  xCentroidOverride/1 -> Mux2/1
  yCentroidOverride/1 -> Mux2/2
  densityThreshold/1 -> Mux3/2
  minPts/1 -> Mux3/3
  maxPts/1 -> Mux3/4
  Mux3/1 -> Dot_detector_pitch/7(clusteringParameters)
  E/1 -> Mux3/1
  centroidOverrideCommand/1 -> Dot_detector_pitch/5(centroidOverrideCommand)
  locationMethod/1 -> Dot_detector_pitch/3(locationMethod)
  dotConfig/1 -> Dot_detector_pitch/4(dotConfig)
  Dot_detector_pitch/2(r1Img) -> Demux/1
  Dot_detector_pitch/3(r2Img) -> Demux1/1
  Dot_detector_pitch/4(rCentroidImg) -> Demux2/1
  Mux2/1 -> Dot_detector_pitch/6(rCentroidManualOverride)
  allOnOff/1 -> Mux/1
  mainImgFeatures/1 -> Mux/2
  mainImgBox/1 -> Mux/3
  mainImgCrosshairs/1 -> Mux/4
  threshInset/1 -> Mux/5
  threshCrosshairs/1 -> Mux/6
  Unused1/1 -> Mux/7
  Unused2/1 -> Mux/8
  Mux/1 -> Dot_detector_pitch/9(viewOptions)
  "u "/1 -> Dot_detector_pitch/1(u)
  Delay13/1 -> Mux1/1
  Delay12/1 -> Mux1/2
  Demux1/1 -> [horiz_centroid_right_y]
  Demux1/2 -> [vert_centroid_right_y]
  Demux/2 -> [vert_centroid_left_y]
  Demux/1 -> [horiz_centroid_left_y]
  Dot_detector_pitch/1(uOut) -> u_out/1
  Demux2/1 -> convertAbsolutePositionToCM/2(xCam), [horiz_centroid_y]
  MATLAB Function/2(x_dist) -> Terminator/1
  MATLAB Function/3(y_dist) -> Terminator3/1
  MATLAB Function/4(z_dist) -> Terminator4/1
  convertPixelsToCM/1(xy) -> xy/1
  convertPixelsToCM/2(yy) -> yy/1
  Demux2/2 -> [vert_centroid_y], convertAbsolutePositionToCM/3(yCam)
  [r_cam] -> convertAbsolutePositionToCM/1(rCam)
  convertAbsolutePositionToCM/1(r) -> rCam3a/1
  view_angle/1 -> [view_angle]
  [view_angle] -> convertAbsolutePositionToCM/4(viewAngle)
  [view_angle] -> convertPixelsToCM/6(viewAngle)
  Mux4/1 -> Dot_detector_pitch/2(roiDims)
  vert_roi_halfwidth/1 -> Mux4/1
  horiz_roi_halfheight/1 -> Mux4/4
  vert_roi_halfheight/1 -> Mux4/2
  horiz_roi_halfwidth/1 -> Mux4/3
  MATLAB Function/1(d_cam_com) -> Saturation1/1
  Saturation1/1 -> Transfer Fcn/1
  Transfer Fcn/1 -> Saturation2/1
  Saturation2/1 -> d_cam/1, convertAbsolutePositionToCM/5(d), convertPixelsToCM/1(d)
  [horiz_centroid_right_y] -> convertPixelsToCM/3(xRight)
  [horiz_centroid_left_y] -> convertPixelsToCM/2(xLeft)
  [vert_centroid_left_y] -> convertPixelsToCM/4(yLeft)
  [vert_centroid_right_y] -> convertPixelsToCM/5(yRight)
  r_cam/1 -> [r_cam], MATLAB Function/1(r_cam)
  "r_com "/1 -> MATLAB Function/2(r_com)

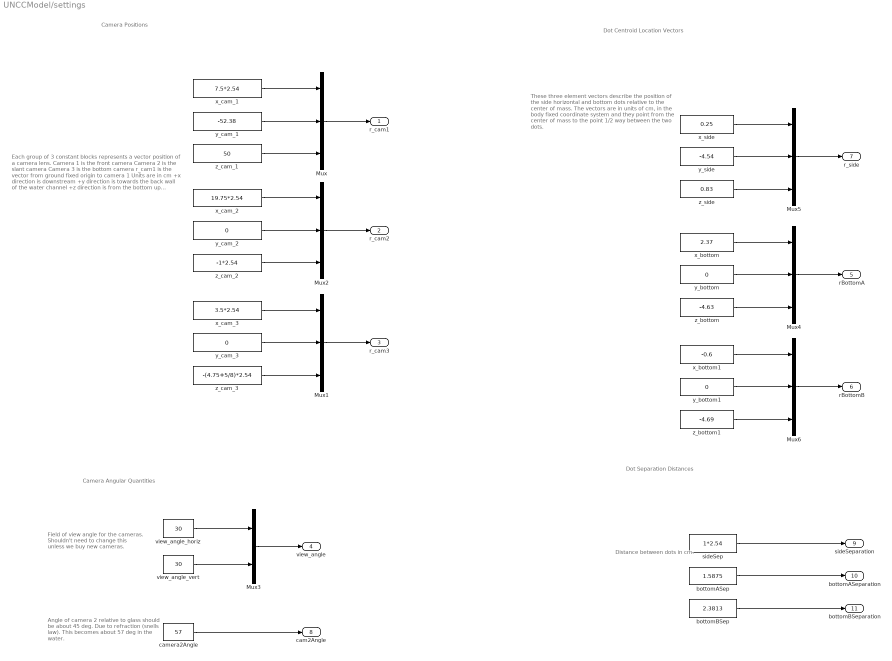
== system UNCCModel/settings ==
  note: Field of view angle
      | for the cameras.
      | Shouldn't need to change
      | this unless we buy new cameras.
  note: Camera Angular Quantities
  note: Dot Separation Distances
  note: Dot Centroid Location Vectors
  note: Camera Positions
  note: Distance between dots
      | in cm.
  note: Angle of camera 2 relative to glass
      | should be about 45 deg.
      |
      | Due to refraction (snells law).  This becomes about 57  deg in the water.
  note: These three element vectors describe the
      | position of the side horizontal and bottom dots
      | relative to the center of mass.  The vectors are in
      | units of cm, in the body fixed coordinate system and
      | they point from the center of mass to the point 1/2
      | way between the two dots.
  note: Each group of 3 constant
      | blocks represents a vector position of a camera lens.
      |
      | Camera 1 is the front camera
      | Camera 2 is the slant camera
      | Camera 3 is the bottom camera
      |
      | r_cam1 is the vector from ground fixed origin to camera 1
      |
      | Units are in cm
      | +x direction is downstream
      | +y direction is towards the back wall of the water channel
      | +z direction is from the bottom up towards the water surface
      |
      | GLASS THICKNESS:
      | Bottom glass: 5/8 in
      | Side glass: 1/2 in
  Mux{,1..2,4..6} (6 alike) : Mux  Inputs=3
  Mux3 : Mux  Inputs=2
  bottomASep : Constant  Value=1.5875
  bottomBSep : Constant  Value=2.3813
  camera2Angle : Constant  Value=57
  sideSep : Constant  Value=1*2.54
  view_angle_horiz : Constant  Value=30
  view_angle_vert : Constant  Value=30
  x_bottom : Constant  Value=2.37
  x_bottom1 : Constant  Value=-0.6
  x_cam_1 : Constant  Value=7.5*2.54
  x_cam_2 : Constant  Value=19.75*2.54
  x_cam_3 : Constant  Value=3.5*2.54
  x_side : Constant  Value=0.25
  y_bottom : Constant  Value=0
  y_bottom1 : Constant  Value=0
  y_cam_1 : Constant  Value=-52.38
  y_cam_2 : Constant  Value=0
  y_cam_3 : Constant  Value=0
  y_side : Constant  Value=-4.54
  z_bottom : Constant  Value=-4.63
  z_bottom1 : Constant  Value=-4.69
  z_cam_1 : Constant  Value=50
  z_cam_2 : Constant  Value=-1*2.54
  z_cam_3 : Constant  Value=-(4.75+5/8)*2.54
  z_side : Constant  Value=0.83
  r_cam1 : Outport
  "r_cam2 " : Outport  Port=2
  r_cam3 : Outport  Port=3
  view_angle : Outport  Port=4
  rBottomA : Outport  Port=5
  rBottomB : Outport  Port=6
  r_side : Outport  Port=7
  cam2Angle : Outport  Port=8
  sideSeparation : Outport  Port=9
  bottomASeparation : Outport  Port=10
  bottomBSeparation : Outport  Port=11
  wires:
  x_cam_1/1 -> Mux/1
  y_cam_1/1 -> Mux/2
  z_cam_1/1 -> Mux/3
  Mux/1 -> r_cam1/1
  x_cam_2/1 -> Mux2/1
  y_cam_2/1 -> Mux2/2
  z_cam_2/1 -> Mux2/3
  x_cam_3/1 -> Mux1/1
  y_cam_3/1 -> Mux1/2
  z_cam_3/1 -> Mux1/3
  Mux2/1 -> "r_cam2 "/1
  Mux1/1 -> r_cam3/1
  view_angle_horiz/1 -> Mux3/1
  view_angle_vert/1 -> Mux3/2
  Mux3/1 -> view_angle/1
  y_bottom/1 -> Mux4/2
  z_bottom/1 -> Mux4/3
  Mux4/1 -> rBottomA/1
  x_bottom/1 -> Mux4/1
  y_side/1 -> Mux5/2
  z_side/1 -> Mux5/3
  Mux5/1 -> r_side/1
  x_side/1 -> Mux5/1
  camera2Angle/1 -> cam2Angle/1
  y_bottom1/1 -> Mux6/2
  z_bottom1/1 -> Mux6/3
  Mux6/1 -> rBottomB/1
  x_bottom1/1 -> Mux6/1
  bottomASep/1 -> bottomASeparation/1
  bottomBSep/1 -> bottomBSeparation/1
  sideSep/1 -> sideSeparation/1
